simulink model "psfb_converter"  (R2024b)
settings: Solver=VariableStepAuto  StartTime=0.0  StopTime=.1  RelTol=1e-3
libraries: spsDiodeLib x4, spsMosfetLib x4, spsSeriesRLCBranchLib x3, spsVoltageMeasurementLib x3, spsCurrentMeasurementLib x2, spsDCVoltageSourceLib x1, spsGroundLib x1, spsLinearTransformerLib x1, sps_lib x1
settings Model: Creator=Yadu  LastModifiedBy=Yadu

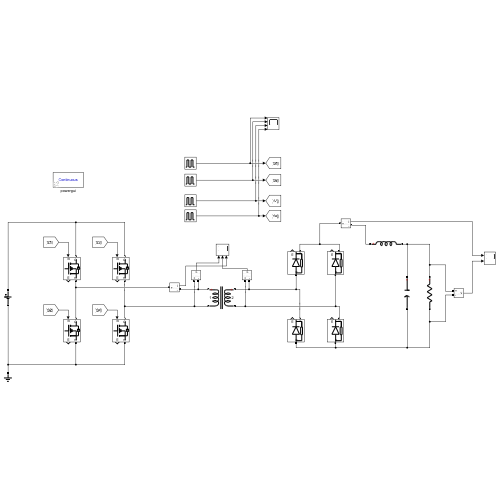
[thumbnail: Simulink's stored preview of the top-level diagram]
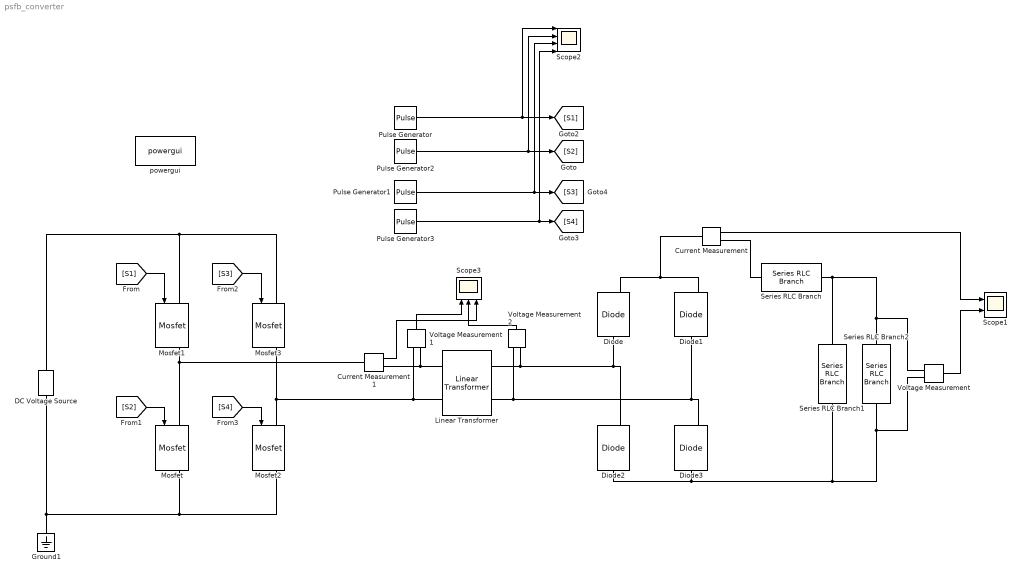
== system psfb_converter ==
  Current Measurement : spsCurrentMeasurementLib/Current Measurement  PhasorSimulation=off  OutputType=Complex  PSBequivalent=0
  Current Measurement1 : spsCurrentMeasurementLib/Current Measurement  PhasorSimulation=off  OutputType=Complex  PSBequivalent=0
  DC Voltage Source : spsDCVoltageSourceLib/DC Voltage Source  Amplitude=120  Measurements=None
  Diode{,1..3} (4 alike) : spsDiodeLib/Diode  Ron=0.001  Lon=0  Vf=0.8  IC=0  UseSnubber=0  Rs=500  Cs=250e-9  Measurements=on
  Ground1 : spsGroundLib/Ground  LConnTagsString=a
  Linear Transformer : spsLinearTransformerLib/Linear Transformer  UNITS=SI  NominalPower=[ 100 200000 ]  winding1=[120 4.3218e-9 0.45856e-9]  winding2=[60 0.7938e-9 0.084225e-9]  ThreeWindings=off  winding3=[3.15e+05 0.7938 0.084225]  RmLm=[1.0804e+06 2866]  Measurements=None  DataType=on
  Mosfet{,1..3} (4 alike) : spsMosfetLib/Mosfet  Ron=0.1  Lon=0  Rd=0.01  Vfd=0  IC=0  Rs=1e5  Cs=inf  Measurements=on
  Pulse Generator : DiscretePulseGenerator  PulseType=Time based  Period=0.000005  PulseWidth=42  PhaseDelay=.0000002125
  Pulse Generator1 : DiscretePulseGenerator  PulseType=Time based  Period=0.000005  PulseWidth=42  PhaseDelay=.0000027125
  Pulse Generator2 : DiscretePulseGenerator  PulseType=Time based  Period=0.000005  PulseWidth=42  PhaseDelay=.0000027125
  Pulse Generator3 : DiscretePulseGenerator  PulseType=Time based  Period=0.000005  PulseWidth=42  PhaseDelay=.0000002125
  Scope1 : Scope  NumInputPorts=2
  Scope2 : Scope  NumInputPorts=4
  Scope3 : Scope  NumInputPorts=3
  Series RLC Branch : spsSeriesRLCBranchLib/Series RLC Branch  LConnTagsString=__new0  RConnTagsString=__new0  BranchType=L  Resistance=1  Inductance=1e-3  SetiL0=off  InitialCurrent=0  Capacitance=1e-6  Setx0=off  InitialVoltage=0  Measurements=None
  Series RLC Branch1 : spsSeriesRLCBranchLib/Series RLC Branch  LConnTagsString=__new0  RConnTagsString=__new0  BranchType=C  Resistance=1  Inductance=1e-3  SetiL0=off  InitialCurrent=0  Capacitance=60e-6  Setx0=off  InitialVoltage=0  Measurements=None
  Series RLC Branch2 : spsSeriesRLCBranchLib/Series RLC Branch  LConnTagsString=__new0  RConnTagsString=__new0  BranchType=R  Resistance=41.66  Inductance=1e-3  SetiL0=off  InitialCurrent=0  Capacitance=1e-6  Setx0=off  InitialVoltage=0  Measurements=None
  Voltage Measurement : spsVoltageMeasurementLib/Voltage Measurement  PhasorSimulation=off  OutputType=Complex  PSBequivalent=0
  Voltage Measurement1 : spsVoltageMeasurementLib/Voltage Measurement  PhasorSimulation=off  OutputType=Complex  PSBequivalent=0
  Voltage Measurement2 : spsVoltageMeasurementLib/Voltage Measurement  PhasorSimulation=off  OutputType=Complex  PSBequivalent=0
  powergui : sps_lib/powergui  Priority=1  SimulationMode=Continuous  SampleTime=50e-6  frequency=60  Iterations=50  frequencyindice=0  Pbase=100e6  ErrMax=1e-4  UnitsV=kV  UnitsW=MW  buscounter=0  FunctionMessages=off  echomessages=off  EnableUseOfTLC=off  CurrentSourceSwitches=off  DisableSnubberDevices=off  DisableRonSwitches=off  DisableVfSwitches=off  DisplayEquations=off  AutomaticDiscreteSolvers=off  SolverType=Tustin/Backward Euler (TBE)  Interpol=off  ExternalGateDelay=off  methode=off  Ts=100  x0status=blocks  SPID=on  SwTol=0  HookPort=off  NonlinearTolerance=1e-4  nMaxIteration=100  ContinueOnMaxIteration=off  RestoreLinks=warning  ResistiveCurrentMeasurement=off  Frange=[0:2:500]  Ylog=off  Xlog=on  ShowGrid=off  save=off  variable=ZData  structure=0  ZoomFFT=off  StartTime=0.0  cycles=1  DisplayStyle=1  fundamental=60  FreqAxis=off  MaxFrequency=1000  frequencyindicesteady=1  RmsSteady=1  display=off
  wires:
  [S4] -> Mosfet2/1
  [S3] -> Mosfet3/1
  [S1] -> Mosfet1/1
  [S2] -> Mosfet/1
  Pulse Generator/1 -> Scope2/1, [S1]
  Pulse Generator3/1 -> Scope2/4, [S4]
  Pulse Generator1/1 -> Scope2/3, [S3]
  Pulse Generator2/1 -> Scope2/2, [S2]
  Current Measurement/1 -> Scope1/1
  Voltage Measurement/1 -> Scope1/2
  Voltage Measurement1/1 -> Scope3/1
  Voltage Measurement2/1 -> Scope3/2
  Current Measurement1/1 -> Scope3/3
  connections:
  Mosfet1/RConn1 -- Current Measurement1/LConn1 -- Mosfet/LConn1
  Mosfet3/LConn1 -- Mosfet1/LConn1 -- DC Voltage Source/RConn1
  Mosfet3/RConn1 -- Voltage Measurement1/LConn1 -- Linear Transformer/LConn2 -- Mosfet2/LConn1
  Mosfet/RConn1 -- DC Voltage Source/LConn1 -- Ground1/LConn1 -- Mosfet2/RConn1
  Linear Transformer/RConn1 -- Voltage Measurement2/LConn2 -- Diode2/RConn1 -- Diode/LConn1
  Diode1/LConn1 -- Diode3/RConn1 -- Linear Transformer/RConn2 -- Voltage Measurement2/LConn1
  Diode1/RConn1 -- Current Measurement/LConn1 -- Diode/RConn1
  Series RLC Branch1/RConn1 -- Diode2/LConn1 -- Diode3/LConn1 -- Series RLC Branch2/RConn1 -- Voltage Measurement/LConn2
  Series RLC Branch1/LConn1 -- Voltage Measurement/LConn1 -- Series RLC Branch2/LConn1 -- Series RLC Branch/RConn1
  Voltage Measurement1/LConn2 -- Linear Transformer/LConn1 -- Current Measurement1/RConn1
  Series RLC Branch/LConn1 -- Current Measurement/RConn1
